simulink model "controllo_cartesiano"  (R2020b)
settings: Solver=VariableStepAuto  StartTime=0.0  StopTime=10.0  RelTol=1e-3
values from neighbouring files (symbols this model uses):
  f_G1 =     [workspaceMassaGravitaCoriolis.mat]
  f_G2 =     [workspaceMassaGravitaCoriolis.mat]
  f_G3 =     [workspaceMassaGravitaCoriolis.mat]
  f_M11 =     [workspaceMassaGravitaCoriolis.mat]
  f_M12 =     [workspaceMassaGravitaCoriolis.mat]
  f_M13 =     [workspaceMassaGravitaCoriolis.mat]
  f_M21 =     [workspaceMassaGravitaCoriolis.mat]
  f_M22 =     [workspaceMassaGravitaCoriolis.mat]
  f_M23 =     [workspaceMassaGravitaCoriolis.mat]
  f_M31 =     [workspaceMassaGravitaCoriolis.mat]
  f_M32 =     [workspaceMassaGravitaCoriolis.mat]
  f_M33 =     [workspaceMassaGravitaCoriolis.mat]
  f_V1 =     [workspaceMassaGravitaCoriolis.mat]
  f_V2 =     [workspaceMassaGravitaCoriolis.mat]
  f_V3 =     [workspaceMassaGravitaCoriolis.mat]
libraries: robotcorelib x1
(part 1 of 5)
settings Model: Creator=frasi  LastModifiedBy=frasi

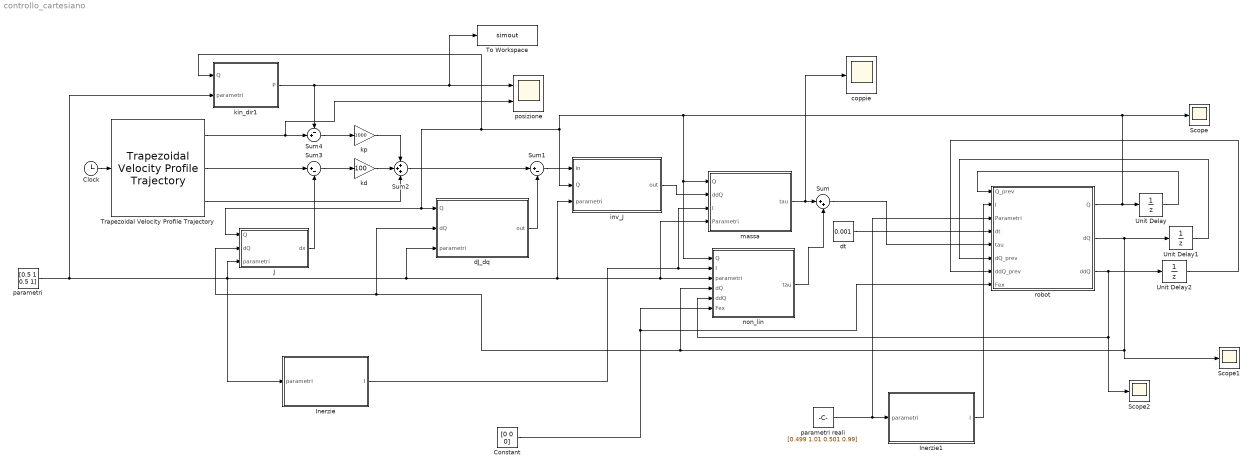
== system controllo_cartesiano ==
  Clock : Clock
  Constant : Constant  Value=[0 0 0]
  Inerzie : MATLAB Function  TreatAsAtomicUnit=on
  Inerzie1 : MATLAB Function  TreatAsAtomicUnit=on
  J : MATLAB Function  TreatAsAtomicUnit=on
  Scope : Scope
  Scope1 : Scope
  Scope2 : Scope
  Sum : Sum  Inputs=|++
  Sum1 : Sum  Inputs=|+-
  Sum2 : Sum  Inputs=+++
  Sum3 : Sum  Inputs=|+-
  Sum4 : Sum  Inputs=-+|
  To Workspace : ToWorkspace  VariableName=simout  SaveFormat=Timeseries  SampleTime=-1
  Trapezoidal Velocity Profile Trajectory : robotcorelib/Trapezoidal Velocity Profile Trajectory  WaypointSource=Internal  Waypoints=[1 1.5; 1.5 2;pi/6 pi/4]  NumParams=1  Parameter1=End Time  Parameter2=Peak Velocity  ParameterSource=Internal  PeakVelocity=[ 4;4 ]  Acceleration=[ 8; 8 ]  EndTime=[ 1; 1 ]  AccelTime=[ 1; 2 ]  SimulateUsing=Interpreted execution
      settings: SourceProductBaseCode=NV,RO,RR,UV
  Unit Delay : UnitDelay  InitialCondition="[0.2403    2.6314    0.9562]"  SampleTime=-1  HasFrameUpgradeWarning=on
  Unit Delay1 : UnitDelay  InitialCondition=[0 0 0]  SampleTime=-1  HasFrameUpgradeWarning=on
  Unit Delay2 : UnitDelay  InitialCondition=[0 0 0]  SampleTime=-1  HasFrameUpgradeWarning=on
  coppie : Scope
  dJ_dq : MATLAB Function  TreatAsAtomicUnit=on
  dt : Constant  Value=0.001
  inv_J : MATLAB Function  TreatAsAtomicUnit=on
  kd : Gain  Gain=100
  kin_dir1 : MATLAB Function  TreatAsAtomicUnit=on
  kp : Gain  Gain=1000
  massa : Subsystem
  non_lin : Subsystem
  parametri : Constant  Value=[0.5 1 0.5 1]
  parametri reali : Constant  Value=[0.499 1.01 0.501 0.99]
  posizione : Scope  NumInputPorts=2
  robot : Subsystem
  wires:
  Trapezoidal Velocity Profile Trajectory/3 -> Sum2/3
  Sum/1 -> robot/5(tau)
  dt/1 -> robot/4(dt)
  kp/1 -> Sum2/1
  Sum3/1 -> kd/1
  Trapezoidal Velocity Profile Trajectory/2 -> Sum3/1
  Sum4/1 -> kp/1
  J/1(dx) -> Sum3/2
  kin_dir1/1(P) -> Sum4/1, To Workspace/1, posizione/1
  Sum1/1 -> inv_J/1(in)
  Sum2/1 -> Sum1/1
  robot/2(dQ) -> Unit Delay1/1, Scope1/1, non_lin/4(dQ), J/2(dQ), dJ_dq/2(dQ)
  non_lin/1(tau) -> Sum/2
  parametri reali/1 -> Inerzie1/1(parametri), robot/3(Parametri)
  parametri/1 -> kin_dir1/2(parametri), inv_J/3(parametri), massa/4(Parametri), non_lin/3(parametri), dJ_dq/3(parametri), Inerzie/1(parametri), J/3(parametri)
  Trapezoidal Velocity Profile Trajectory/1 -> posizione/2, Sum4/2
  kd/1 -> Sum2/2
  massa/1(tau) -> coppie/1, Sum/1
  robot/1(Q) -> non_lin/1(Q), massa/1(Q), kin_dir1/1(Q), J/1(Q), dJ_dq/1(Q), inv_J/2(Q), Scope/1, Unit Delay/1
  Clock/1 -> Trapezoidal Velocity Profile Trajectory/1
  dJ_dq/1(out) -> Sum1/2
  Unit Delay/1 -> robot/1(Q_prev)
  Unit Delay1/1 -> robot/6(dQ_prev)
  inv_J/1(out) -> massa/2(ddQ)
  robot/3(ddQ) -> Unit Delay2/1, Scope2/1, non_lin/5(ddQ)
  Unit Delay2/1 -> robot/7(ddQ_prev)
  Inerzie/1(I) -> massa/3(I), non_lin/2(I)
  Inerzie1/1(I) -> robot/2(I)
  Constant/1 -> non_lin/6(Fex), robot/8(Fex)

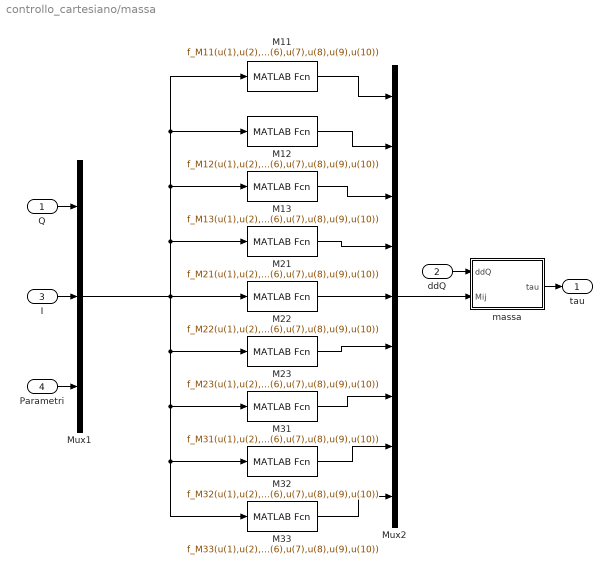
== system controllo_cartesiano/massa ==
  Q : Inport
  ddQ : Inport  Port=2
  I : Inport  Port=3
  Parametri : Inport  Port=4
  M11 : MATLABFcn  MATLABFcn=f_M11(u(1),u(2),u(3),u(4),u(5),u(6),u(7),u(8),u(9),u(10))
  M12 : MATLABFcn  MATLABFcn=f_M12(u(1),u(2),u(3),u(4),u(5),u(6),u(7),u(8),u(9),u(10))
  M13 : MATLABFcn  MATLABFcn=f_M13(u(1),u(2),u(3),u(4),u(5),u(6),u(7),u(8),u(9),u(10))
  M21 : MATLABFcn  MATLABFcn=f_M21(u(1),u(2),u(3),u(4),u(5),u(6),u(7),u(8),u(9),u(10))
  M22 : MATLABFcn  MATLABFcn=f_M22(u(1),u(2),u(3),u(4),u(5),u(6),u(7),u(8),u(9),u(10))
  M23 : MATLABFcn  MATLABFcn=f_M23(u(1),u(2),u(3),u(4),u(5),u(6),u(7),u(8),u(9),u(10))
  M31 : MATLABFcn  MATLABFcn=f_M31(u(1),u(2),u(3),u(4),u(5),u(6),u(7),u(8),u(9),u(10))
  M32 : MATLABFcn  MATLABFcn=f_M32(u(1),u(2),u(3),u(4),u(5),u(6),u(7),u(8),u(9),u(10))
  M33 : MATLABFcn  MATLABFcn=f_M33(u(1),u(2),u(3),u(4),u(5),u(6),u(7),u(8),u(9),u(10))
  Mux1 : Mux  Inputs=3
  Mux2 : Mux  Inputs=9
  massa : MATLAB Function  TreatAsAtomicUnit=on
  tau : Outport
  wires:
  M13/1 -> Mux2/3
  Mux2/1 -> massa/2(Mij)
  M33/1 -> Mux2/9
  M11/1 -> Mux2/1
  Mux1/1 -> M13/1, M12/1, M11/1, M21/1, M31/1, M32/1, M33/1, M23/1, M22/1
  M22/1 -> Mux2/5
  M23/1 -> Mux2/6
  M31/1 -> Mux2/7
  M21/1 -> Mux2/4
  M12/1 -> Mux2/2
  Parametri/1 -> Mux1/3
  M32/1 -> Mux2/8
  ddQ/1 -> massa/1(ddQ)
  I/1 -> Mux1/2
  Q/1 -> Mux1/1
  massa/1(tau) -> tau/1

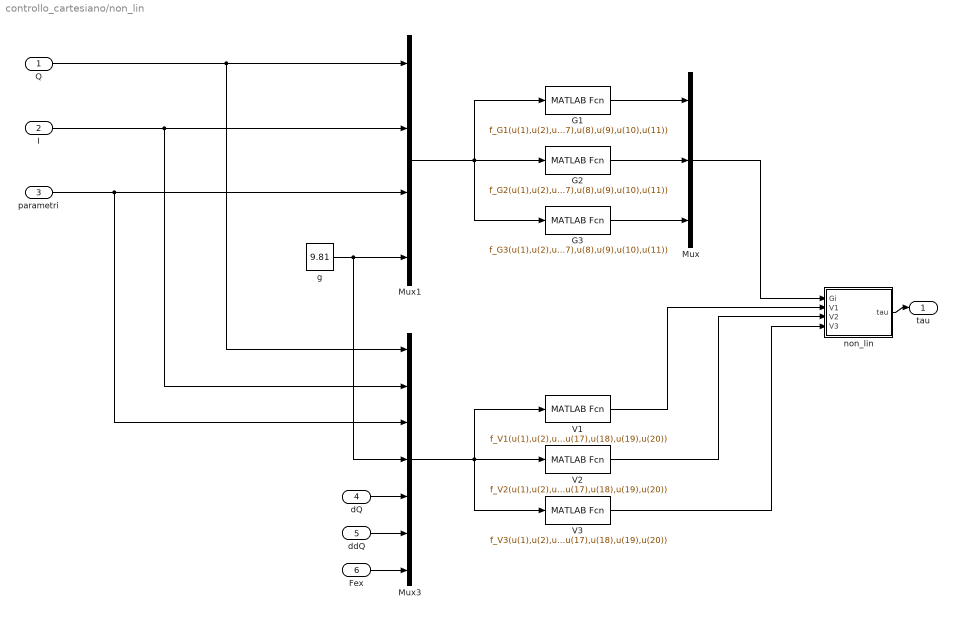
== system controllo_cartesiano/non_lin ==
  Q : Inport
  I : Inport  Port=2
  parametri : Inport  Port=3
  dQ : Inport  Port=4
  ddQ : Inport  Port=5
  Fex : Inport  Port=6
  G1 : MATLABFcn  MATLABFcn=f_G1(u(1),u(2),u(3),u(4),u(5),u(6),u(7),u(8),u(9),u(10),u(11))
  G2 : MATLABFcn  MATLABFcn=f_G2(u(1),u(2),u(3),u(4),u(5),u(6),u(7),u(8),u(9),u(10),u(11))
  G3 : MATLABFcn  MATLABFcn=f_G3(u(1),u(2),u(3),u(4),u(5),u(6),u(7),u(8),u(9),u(10),u(11))
  Mux : Mux  Inputs=3
  Mux1 : Mux
  Mux3 : Mux  Inputs=7
  V1 : MATLABFcn  MATLABFcn=f_V1(u(1),u(2),u(3),u(4),u(5),u(6),u(7),u(8),u(9),u(10),u(11),u(12),u(13),u(14),u(15),u(16),u(17),u(18),u(19),u(20))
  V2 : MATLABFcn  MATLABFcn=f_V2(u(1),u(2),u(3),u(4),u(5),u(6),u(7),u(8),u(9),u(10),u(11),u(12),u(13),u(14),u(15),u(16),u(17),u(18),u(19),u(20))
  V3 : MATLABFcn  MATLABFcn=f_V3(u(1),u(2),u(3),u(4),u(5),u(6),u(7),u(8),u(9),u(10),u(11),u(12),u(13),u(14),u(15),u(16),u(17),u(18),u(19),u(20))
  g : Constant  Value=9.81
  non_lin : MATLAB Function  TreatAsAtomicUnit=on
  tau : Outport
  wires:
  Mux3/1 -> V3/1, V2/1, V1/1
  g/1 -> Mux3/4, Mux1/4
  parametri/1 -> Mux3/3, Mux1/3
  Mux1/1 -> G3/1, G2/1, G1/1
  non_lin/1(tau) -> tau/1
  Q/1 -> Mux3/1, Mux1/1
  Fex/1 -> Mux3/7
  I/1 -> Mux3/2, Mux1/2
  dQ/1 -> Mux3/5
  ddQ/1 -> Mux3/6
  V1/1 -> non_lin/2(V1)
  V2/1 -> non_lin/3(V2)
  V3/1 -> non_lin/4(V3)
  Mux/1 -> non_lin/1(Gi)
  G1/1 -> Mux/1
  G2/1 -> Mux/2
  G3/1 -> Mux/3

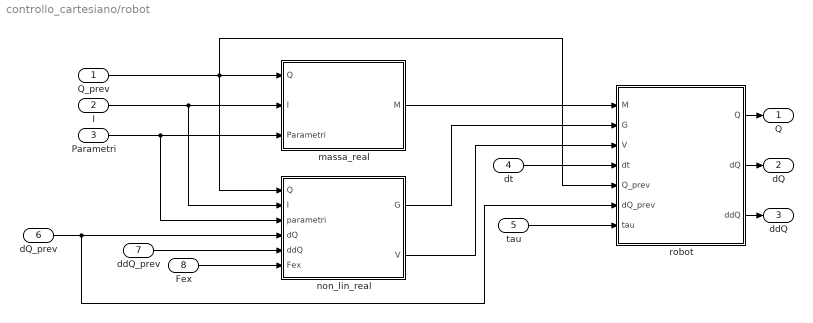
== system controllo_cartesiano/robot ==
  Q_prev : Inport
  I : Inport  Port=2
  Parametri : Inport  Port=3
  dt : Inport  Port=4
  tau : Inport  Port=5
  dQ_prev : Inport  Port=6
  ddQ_prev : Inport  Port=7
  Fex : Inport  Port=8
  massa_real : Subsystem
  non_lin_real : Subsystem
  robot : MATLAB Function  TreatAsAtomicUnit=on
  Q : Outport
  dQ : Outport  Port=2
  ddQ : Outport  Port=3
  wires:
  Parametri/1 -> non_lin_real/3(parametri), massa_real/3(Parametri)
  non_lin_real/1(G) -> robot/2(G)
  ddQ_prev/1 -> non_lin_real/5(ddQ)
  Fex/1 -> non_lin_real/6(Fex)
  non_lin_real/2(V) -> robot/3(V)
  I/1 -> non_lin_real/2(I), massa_real/2(I)
  massa_real/1(M) -> robot/1(M)
  robot/1(Q) -> Q/1
  Q_prev/1 -> robot/5(Q_prev), massa_real/1(Q), non_lin_real/1(Q)
  dQ_prev/1 -> robot/6(dQ_prev), non_lin_real/4(dQ)
  tau/1 -> robot/7(tau)
  robot/2(dQ) -> dQ/1
  dt/1 -> robot/4(dt)
  robot/3(ddQ) -> ddQ/1

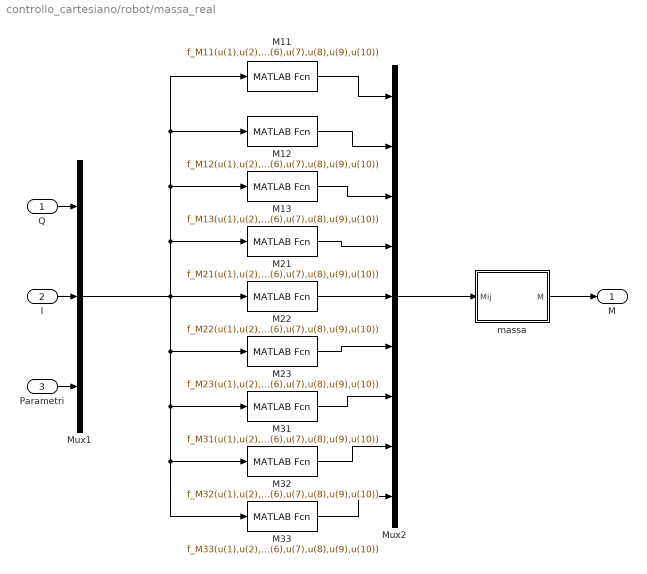
== system controllo_cartesiano/robot/massa_real ==
  Q : Inport
  I : Inport  Port=2
  Parametri : Inport  Port=3
  M11 : MATLABFcn  MATLABFcn=f_M11(u(1),u(2),u(3),u(4),u(5),u(6),u(7),u(8),u(9),u(10))
  M12 : MATLABFcn  MATLABFcn=f_M12(u(1),u(2),u(3),u(4),u(5),u(6),u(7),u(8),u(9),u(10))
  M13 : MATLABFcn  MATLABFcn=f_M13(u(1),u(2),u(3),u(4),u(5),u(6),u(7),u(8),u(9),u(10))
  M21 : MATLABFcn  MATLABFcn=f_M21(u(1),u(2),u(3),u(4),u(5),u(6),u(7),u(8),u(9),u(10))
  M22 : MATLABFcn  MATLABFcn=f_M22(u(1),u(2),u(3),u(4),u(5),u(6),u(7),u(8),u(9),u(10))
  M23 : MATLABFcn  MATLABFcn=f_M23(u(1),u(2),u(3),u(4),u(5),u(6),u(7),u(8),u(9),u(10))
  M31 : MATLABFcn  MATLABFcn=f_M31(u(1),u(2),u(3),u(4),u(5),u(6),u(7),u(8),u(9),u(10))
  M32 : MATLABFcn  MATLABFcn=f_M32(u(1),u(2),u(3),u(4),u(5),u(6),u(7),u(8),u(9),u(10))
  M33 : MATLABFcn  MATLABFcn=f_M33(u(1),u(2),u(3),u(4),u(5),u(6),u(7),u(8),u(9),u(10))
  Mux1 : Mux  Inputs=3
  Mux2 : Mux  Inputs=9
  massa : MATLAB Function  TreatAsAtomicUnit=on
  M : Outport
  wires:
  M13/1 -> Mux2/3
  Mux2/1 -> massa/1(Mij)
  M33/1 -> Mux2/9
  M11/1 -> Mux2/1
  Mux1/1 -> M13/1, M12/1, M11/1, M21/1, M31/1, M32/1, M33/1, M23/1, M22/1
  M22/1 -> Mux2/5
  M23/1 -> Mux2/6
  M31/1 -> Mux2/7
  M21/1 -> Mux2/4
  M12/1 -> Mux2/2
  Parametri/1 -> Mux1/3
  M32/1 -> Mux2/8
  I/1 -> Mux1/2
  Q/1 -> Mux1/1
  massa/1(M) -> M/1

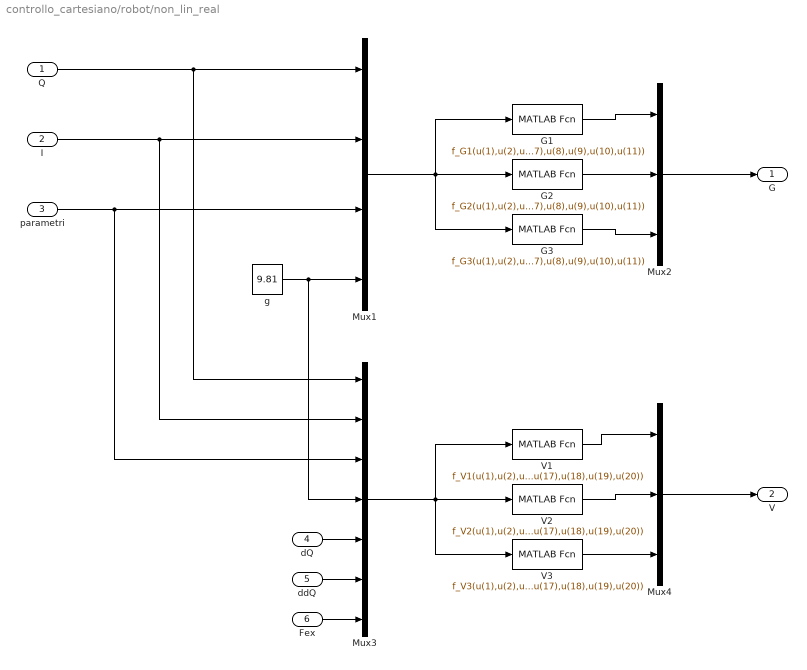
== system controllo_cartesiano/robot/non_lin_real ==
  Q : Inport
  I : Inport  Port=2
  parametri : Inport  Port=3
  dQ : Inport  Port=4
  ddQ : Inport  Port=5
  Fex : Inport  Port=6
  G1 : MATLABFcn  MATLABFcn=f_G1(u(1),u(2),u(3),u(4),u(5),u(6),u(7),u(8),u(9),u(10),u(11))
  G2 : MATLABFcn  MATLABFcn=f_G2(u(1),u(2),u(3),u(4),u(5),u(6),u(7),u(8),u(9),u(10),u(11))
  G3 : MATLABFcn  MATLABFcn=f_G3(u(1),u(2),u(3),u(4),u(5),u(6),u(7),u(8),u(9),u(10),u(11))
  Mux1 : Mux
  Mux2 : Mux  Inputs=3
  Mux3 : Mux  Inputs=7
  Mux4 : Mux  Inputs=3
  V1 : MATLABFcn  MATLABFcn=f_V1(u(1),u(2),u(3),u(4),u(5),u(6),u(7),u(8),u(9),u(10),u(11),u(12),u(13),u(14),u(15),u(16),u(17),u(18),u(19),u(20))
  V2 : MATLABFcn  MATLABFcn=f_V2(u(1),u(2),u(3),u(4),u(5),u(6),u(7),u(8),u(9),u(10),u(11),u(12),u(13),u(14),u(15),u(16),u(17),u(18),u(19),u(20))
  V3 : MATLABFcn  MATLABFcn=f_V3(u(1),u(2),u(3),u(4),u(5),u(6),u(7),u(8),u(9),u(10),u(11),u(12),u(13),u(14),u(15),u(16),u(17),u(18),u(19),u(20))
  g : Constant  Value=9.81
  G : Outport
  V : Outport  Port=2
  wires:
  Mux3/1 -> V3/1, V2/1, V1/1
  g/1 -> Mux3/4, Mux1/4
  V2/1 -> Mux4/2
  G2/1 -> Mux2/2
  Q/1 -> Mux3/1, Mux1/1
  Mux1/1 -> G3/1, G2/1, G1/1
  V3/1 -> Mux4/3
  V1/1 -> Mux4/1
  G1/1 -> Mux2/1
  G3/1 -> Mux2/3
  Mux4/1 -> V/1
  Mux2/1 -> G/1
  parametri/1 -> Mux3/3, Mux1/3
  Fex/1 -> Mux3/7
  I/1 -> Mux3/2, Mux1/2
  ddQ/1 -> Mux3/6
  dQ/1 -> Mux3/5

== matlab function controllo_cartesiano/non_lin/non_lin ==
  data: Gi input; tau output; V1 input; V2 input; V3 input
function tau = non_lin(Gi,V1,V2,V3)

G=[Gi(1);Gi(2);Gi(3)];
V=[V1;V2;V3];

tau=G+V;
end

== matlab function controllo_cartesiano/massa/massa ==
  data: ddQ input; tau output; Mij input
function  tau= massa(ddQ,Mij)

M=[Mij(1) Mij(2) Mij(3);Mij(4) Mij(5) Mij(6);Mij(7) Mij(8) Mij(9)];
tau=M*ddQ;

end

== matlab function controllo_cartesiano/inv_J ==
  data: in input; out output; Q input; parametri input
function out = inv_J(in,Q,parametri)
l=parametri(1);
d=parametri(2);
% m1=parametri(3);
% ma=parametri(4);
xc1=Q(1);
xc5=Q(2);
q2=Q(3);

J =[...
 
(l*sin(2*atan((2*l^2*sin(q2) + (3*l^4 + 4*cos(q2)*l^3*xc1 - 4*sin(q2)*l^3*xc5 - 2*cos(2*q2)*l^2*xc1^2 + 4*sin(2*q2)*l^2*xc1*xc5 + 2*cos(2*q2)*l^2*xc5^2 - 4*cos(q2)*l*xc1^3 + 4*sin(q2)*l*xc1^2*xc5 - 4*cos(q2)*l*xc1*xc5^2 + 4*sin(q2)*l*xc5^3 - xc1^4 - 2*xc1^2*xc5^2 - xc5^4)^(1/2) - 2*l*xc5)/(l^2 - 2*l*xc1 + xc1^2 + xc5^2 - 2*l^2*cos(q2) + 2*l*xc1*cos(q2) - 2*l*xc5*sin(q2))))*(((2*xc1 - 2*l + 2*l*cos(q2))*(2*l^2*sin(q2) + (3*l^4 + 4*cos(q2)*l^3*xc1 - 4*sin(q2)*l^3*xc5 - 2*cos(2*q2)*l^2*xc1^2 + 4*sin(2*q2)*l^2*xc1*xc5 + 2*cos(2*q2)*l^2*xc5^2 - 4*cos(q2)*l*xc1^3 + 4*sin(q2)*l*xc1^2*xc5 - 4*cos(q2)*l*xc1*xc5^2 + 4*sin(q2)*l*xc5^3 - xc1^4 - 2*xc1^2*xc5^2 - xc5^4)^(1/2) - 2*l*xc5))/(l^2 - 2*l*xc1 + xc1^2 + xc5^2 - 2*l^2*cos(q2) + 2*l*xc1*cos(q2) - 2*l*xc5*sin(q2))^2 + (2*(xc1 + l*cos(q2))*(- l^2 + 2*cos(q2)*l*xc1 - 2*sin(q2)*l*xc5 + xc1^2 + xc5^2))/((l^2 - 2*l*xc1 + xc1^2 + xc5^2 - 2*l^2*cos(q2) + 2*l*xc1*cos(q2) - 2*l*xc5*sin(q2))*(3*l^4 + 4*cos(q2)*l^3*xc1 - 4*sin(q2)*l^3*xc5 - 2*cos(2*q2)*l^2*xc1^2 + 4*sin(2*q2)*l^2*xc1*xc5 + 2*cos(2*q2)*l^2*xc5^2 - 4*cos(q2)*l*xc1^3 + 4*sin(q2)*l*xc1^2*xc5 - 4*cos(q2)*l*xc1*xc5^2 + 4*sin(q2)*l*xc5^3 - xc1^4 - 2*xc1^2*xc5^2 - xc5^4)^(1/2))))/((2*l^2*sin(q2) + (3*l^4 + 4*cos(q2)*l^3*xc1 - 4*sin(q2)*l^3*xc5 - 2*cos(2*q2)*l^2*xc1^2 + 4*sin(2*q2)*l^2*xc1*xc5 + 2*cos(2*q2)*l^2*xc5^2 - 4*cos(q2)*l*xc1^3 + 4*sin(q2)*l*xc1^2*xc5 - 4*cos(q2)*l*xc1*xc5^2 + 4*sin(q2)*l*xc5^3 - xc1^4 - 2*xc1^2*xc5^2 - xc5^4)^(1/2) - 2*l*xc5)^2/(l^2 - 2*l*xc1 + xc1^2 + xc5^2 - 2*l^2*cos(q2) + 2*l*xc1*cos(q2) - 2*l*xc5*sin(q2))^2 + 1) + 1, (l*sin(2*atan((2*l^2*sin(q2) + (3*l^4 + 4*cos(q2)*l^3*xc1 - 4*sin(q2)*l^3*xc5 - 2*cos(2*q2)*l^2*xc1^2 + 4*sin(2*q2)*l^2*xc1*xc5 + 2*cos(2*q2)*l^2*xc5^2 - 4*cos(q2)*l*xc1^3 + 4*sin(q2)*l*xc1^2*xc5 - 4*cos(q2)*l*xc1*xc5^2 + 4*sin(q2)*l*xc5^3 - xc1^4 - 2*xc1^2*xc5^2 - xc5^4)^(1/2) - 2*l*xc5)/(l^2 - 2*l*xc1 + xc1^2 + xc5^2 - 2*l^2*cos(q2) + 2*l*xc1*cos(q2) - 2*l*xc5*sin(q2))))*((2*l + (2*sin(q2)*l^3 - 2*sin(2*q2)*l^2*xc1 - 2*cos(2*q2)*l^2*xc5 - 2*sin(q2)*l*xc1^2 + 4*cos(q2)*l*xc1*xc5 - 6*sin(q2)*l*xc5^2 + 2*xc1^2*xc5 + 2*xc5^3)/(3*l^4 + 4*cos(q2)*l^3*xc1 - 4*sin(q2)*l^3*xc5 - 2*cos(2*q2)*l^2*xc1^2 + 4*sin(2*q2)*l^2*xc1*xc5 + 2*cos(2*q2)*l^2*xc5^2 - 4*cos(q2)*l*xc1^3 + 4*sin(q2)*l*xc1^2*xc5 - 4*cos(q2)*l*xc1*xc5^2 + 4*sin(q2)*l*xc5^3 - xc1^4 - 2*xc1^2*xc5^2 - xc5^4)^(1/2))/(l^2 - 2*l*xc1 + xc1^2 + xc5^2 - 2*l^2*cos(q2) + 2*l*xc1*cos(q2) - 2*l*xc5*sin(q2)) + ((2*xc5 - 2*l*sin(q2))*(2*l^2*sin(q2) + (3*l^4 + 4*cos(q2)*l^3*xc1 - 4*sin(q2)*l^3*xc5 - 2*cos(2*q2)*l^2*xc1^2 + 4*sin(2*q2)*l^2*xc1*xc5 + 2*cos(2*q2)*l^2*xc5^2 - 4*cos(q2)*l*xc1^3 + 4*sin(q2)*l*xc1^2*xc5 - 4*cos(q2)*l*xc1*xc5^2 + 4*sin(q2)*l*xc5^3 - xc1^4 - 2*xc1^2*xc5^2 - xc5^4)^(1/2) - 2*l*xc5))/(l^2 - 2*l*xc1 + xc1^2 + xc5^2 - 2*l^2*cos(q2) + 2*l*xc1*cos(q2) - 2*l*xc5*sin(q2))^2))/((2*l^2*sin(q2) + (3*l^4 + 4*cos(q2)*l^3*xc1 - 4*sin(q2)*l^3*xc5 - 2*cos(2*q2)*l^2*xc1^2 + 4*sin(2*q2)*l^2*xc1*xc5 + 2*cos(2*q2)*l^2*xc5^2 - 4*cos(q2)*l*xc1^3 + 4*sin(q2)*l*xc1^2*xc5 - 4*cos(q2)*l*xc1*xc5^2 + 4*sin(q2)*l*xc5^3 - xc1^4 - 2*xc1^2*xc5^2 - xc5^4)^(1/2) - 2*l*xc5)^2/(l^2 - 2*l*xc1 + xc1^2 + xc5^2 - 2*l^2*cos(q2) + 2*l*xc1*cos(q2) - 2*l*xc5*sin(q2))^2 + 1), - l*sin(q2) - (l*sin(2*atan((2*l^2*sin(q2) + (3*l^4 + 4*cos(q2)*l^3*xc1 - 4*sin(q2)*l^3*xc5 - 2*cos(2*q2)*l^2*xc1^2 + 4*sin(2*q2)*l^2*xc1*xc5 + 2*cos(2*q2)*l^2*xc5^2 - 4*cos(q2)*l*xc1^3 + 4*sin(q2)*l*xc1^2*xc5 - 4*cos(q2)*l*xc1*xc5^2 + 4*sin(q2)*l*xc5^3 - xc1^4 - 2*xc1^2*xc5^2 - xc5^4)^(1/2) - 2*l*xc5)/(l^2 - 2*l*xc1 + xc1^2 + xc5^2 - 2*l^2*cos(q2) + 2*l*xc1*cos(q2) - 2*l*xc5*sin(q2))))*((2*l^2*cos(q2) + (2*l*(- sin(q2)*l^2*xc1 - cos(q2)*l^2*xc5 + sin(2*q2)*l*xc1^2 + 2*cos(2*q2)*l*xc1*xc5 - sin(2*q2)*l*xc5^2 + sin(q2)*xc1^3 + cos(q2)*xc1^2*xc5 + sin(q2)*xc1*xc5^2 + cos(q2)*xc5^3))/(3*l^4 + 4*cos(q2)*l^3*xc1 - 4*sin(q2)*l^3*xc5 - 2*cos(2*q2)*l^2*xc1^2 + 4*sin(2*q2)*l^2*xc1*xc5 + 2*cos(2*q2)*l^2*xc5^2 - 4*cos(q2)*l*xc1^3 + 4*sin(q2)*l*xc1^2*xc5 - 4*cos(q2)*l*xc1*xc5^2 + 4*sin(q2)*l*xc5^3 - xc1^4 - 2*xc1^2*xc5^2 - xc5^4)^(1/2))/(l^2 - 2*l*xc1 + xc1^2 + xc5^2 - 2*l^2*cos(q2) + 2*l*xc1*cos(q2) - 2*l*xc5*sin(q2)) + (2*l*(xc5*cos(q2) - l*sin(q2) + xc1*sin(q2))*(2*l^2*sin(q2) + (3*l^4 + 4*cos(q2)*l^3*xc1 - 4*sin(q2)*l^3*xc5 - 2*cos(2*q2)*l^2*xc1^2 + 4*sin(2*q2)*l^2*xc1*xc5 + 2*cos(2*q2)*l^2*xc5^2 - 4*cos(q2)*l*xc1^3 + 4*sin(q2)*l*xc1^2*xc5 - 4*cos(q2)*l*xc1*xc5^2 + 4*sin(q2)*l*xc5^3 - xc1^4 - 2*xc1^2*xc5^2 - xc5^4)^(1/2) - 2*l*xc5))/(l^2 - 2*l*xc1 + xc1^2 + xc5^2 - 2*l^2*cos(q2) + 2*l*xc1*cos(q2) - 2*l*xc5*sin(q2))^2))/((2*l^2*sin(q2) + (3*l^4 + 4*cos(q2)*l^3*xc1 - 4*sin(q2)*l^3*xc5 - 2*cos(2*q2)*l^2*xc1^2 + 4*sin(2*q2)*l^2*xc1*xc5 + 2*cos(2*q2)*l^2*xc5^2 - 4*cos(q2)*l*xc1^3 + 4*sin(q2)*l*xc1^2*xc5 - 4*cos(q2)*l*xc1*xc5^2 + 4*sin(q2)*l*xc5^3 - xc1^4 - 2*xc1^2*xc5^2 - xc5^4)^(1/2) - 2*l*xc5)^2/(l^2 - 2*l*xc1 + xc1^2 + xc5^2 - 2*l^2*cos(q2) + 2*l*xc1*cos(q2) - 2*l*xc5*sin(q2))^2 + 1);...
    (l*cos(2*atan((2*l^2*sin(q2) + (3*l^4 + 4*cos(q2)*l^3*xc1 - 4*sin(q2)*l^3*xc5 - 2*cos(2*q2)*l^2*xc1^2 + 4*sin(2*q2)*l^2*xc1*xc5 + 2*cos(2*q2)*l^2*xc5^2 - 4*cos(q2)*l*xc1^3 + 4*sin(q2)*l*xc1^2*xc5 - 4*cos(q2)*l*xc1*xc5^2 + 4*sin(q2)*l*xc5^3 - xc1^4 - 2*xc1^2*xc5^2 - xc5^4)^(1/2) - 2*l*xc5)/(l^2 - 2*l*xc1 + xc1^2 + xc5^2 - 2*l^2*cos(q2) + 2*l*xc1*cos(q2) - 2*l*xc5*sin(q2))))*(((2*xc1 - 2*l + 2*l*cos(q2))*(2*l^2*sin(q2) + (3*l^4 + 4*cos(q2)*l^3*xc1 - 4*sin(q2)*l^3*xc5 - 2*cos(2*q2)*l^2*xc1^2 + 4*sin(2*q2)*l^2*xc1*xc5 + 2*cos(2*q2)*l^2*xc5^2 - 4*cos(q2)*l*xc1^3 + 4*sin(q2)*l*xc1^2*xc5 - 4*cos(q2)*l*xc1*xc5^2 + 4*sin(q2)*l*xc5^3 - xc1^4 - 2*xc1^2*xc5^2 - xc5^4)^(1/2) - 2*l*xc5))/(l^2 - 2*l*xc1 + xc1^2 + xc5^2 - 2*l^2*cos(q2) + 2*l*xc1*cos(q2) - 2*l*xc5*sin(q2))^2 + (2*(xc1 + l*cos(q2))*(- l^2 + 2*cos(q2)*l*xc1 - 2*sin(q2)*l*xc5 + xc1^2 + xc5^2))/((l^2 - 2*l*xc1 + xc1^2 + xc5^2 - 2*l^2*cos(q2) + 2*l*xc1*cos(q2) - 2*l*xc5*sin(q2))*(3*l^4 + 4*cos(q2)*l^3*xc1 - 4*sin(q2)*l^3*xc5 - 2*cos(2*q2)*l^2*xc1^2 + 4*sin(2*q2)*l^2*xc1*xc5 + 2*cos(2*q2)*l^2*xc5^2 - 4*cos(q2)*l*xc1^3 + 4*sin(q2)*l*xc1^2*xc5 - 4*cos(q2)*l*xc1*xc5^2 + 4*sin(q2)*l*xc5^3 - xc1^4 - 2*xc1^2*xc5^2 - xc5^4)^(1/2))))/((2*l^2*sin(q2) + (3*l^4 + 4*cos(q2)*l^3*xc1 - 4*sin(q2)*l^3*xc5 - 2*cos(2*q2)*l^2*xc1^2 + 4*sin(2*q2)*l^2*xc1*xc5 + 2*cos(2*q2)*l^2*xc5^2 - 4*cos(q2)*l*xc1^3 + 4*sin(q2)*l*xc1^2*xc5 - 4*cos(q2)*l*xc1*xc5^2 + 4*sin(q2)*l*xc5^3 - xc1^4 - 2*xc1^2*xc5^2 - xc5^4)^(1/2) - 2*l*xc5)^2/(l^2 - 2*l*xc1 + xc1^2 + xc5^2 - 2*l^2*cos(q2) + 2*l*xc1*cos(q2) - 2*l*xc5*sin(q2))^2 + 1), (l*cos(2*atan((2*l^2*sin(q2) + (3*l^4 + 4*cos(q2)*l^3*xc1 - 4*sin(q2)*l^3*xc5 - 2*cos(2*q2)*l^2*xc1^2 + 4*sin(2*q2)*l^2*xc1*xc5 + 2*cos(2*q2)*l^2*xc5^2 - 4*cos(q2)*l*xc1^3 + 4*sin(q2)*l*xc1^2*xc5 - 4*cos(q2)*l*xc1*xc5^2 + 4*sin(q2)*l*xc5^3 - xc1^4 - 2*xc1^2*xc5^2 - xc5^4)^(1/2) - 2*l*xc5)/(l^2 - 2*l*xc1 + xc1^2 + xc5^2 - 2*l^2*cos(q2) + 2*l*xc1*cos(q2) - 2*l*xc5*sin(q2))))*((2*l + (2*sin(q2)*l^3 - 2*sin(2*q2)*l^2*xc1 - 2*cos(2*q2)*l^2*xc5 - 2*sin(q2)*l*xc1^2 + 4*cos(q2)*l*xc1*xc5 - 6*sin(q2)*l*xc5^2 + 2*xc1^2*xc5 + 2*xc5^3)/(3*l^4 + 4*cos(q2)*l^3*xc1 - 4*sin(q2)*l^3*xc5 - 2*cos(2*q2)*l^2*xc1^2 + 4*sin(2*q2)*l^2*xc1*xc5 + 2*cos(2*q2)*l^2*xc5^2 - 4*cos(q2)*l*xc1^3 + 4*sin(q2)*l*xc1^2*xc5 - 4*cos(q2)*l*xc1*xc5^2 + 4*sin(q2)*l*xc5^3 - xc1^4 - 2*xc1^2*xc5^2 - xc5^4)^(1/2))/(l^2 - 2*l*xc1 + xc1^2 + xc5^2 - 2*l^2*cos(q2) + 2*l*xc1*cos(q2) - 2*l*xc5*sin(q2)) + ((2*xc5 - 2*l*sin(q2))*(2*l^2*sin(q2) + (3*l^4 + 4*cos(q2)*l^3*xc1 - 4*sin(q2)*l^3*xc5 - 2*cos(2*q2)*l^2*xc1^2 + 4*sin(2*q2)*l^2*xc1*xc5 + 2*cos(2*q2)*l^2*xc5^2 - 4*cos(q2)*l*xc1^3 + 4*sin(q2)*l*xc1^2*xc5 - 4*cos(q2)*l*xc1*xc5^2 + 4*sin(q2)*l*xc5^3 - xc1^4 - 2*xc1^2*xc5^2 - xc5^4)^(1/2) - 2*l*xc5))/(l^2 - 2*l*xc1 + xc1^2 + xc5^2 - 2*l^2*cos(q2) + 2*l*xc1*cos(q2) - 2*l*xc5*sin(q2))^2))/((2*l^2*sin(q2) + (3*l^4 + 4*cos(q2)*l^3*xc1 - 4*sin(q2)*l^3*xc5 - 2*cos(2*q2)*l^2*xc1^2 + 4*sin(2*q2)*l^2*xc1*xc5 + 2*cos(2*q2)*l^2*xc5^2 - 4*cos(q2)*l*xc1^3 + 4*sin(q2)*l*xc1^2*xc5 - 4*cos(q2)*l*xc1*xc5^2 + 4*sin(q2)*l*xc5^3 - xc1^4 - 2*xc1^2*xc5^2 - xc5^4)^(1/2) - 2*l*xc5)^2/(l^2 - 2*l*xc1 + xc1^2 + xc5^2 - 2*l^2*cos(q2) + 2*l*xc1*cos(q2) - 2*l*xc5*sin(q2))^2 + 1),   l*cos(q2) - (l*cos(2*atan((2*l^2*sin(q2) + (3*l^4 + 4*cos(q2)*l^3*xc1 - 4*sin(q2)*l^3*xc5 - 2*cos(2*q2)*l^2*xc1^2 + 4*sin(2*q2)*l^2*xc1*xc5 + 2*cos(2*q2)*l^2*xc5^2 - 4*cos(q2)*l*xc1^3 + 4*sin(q2)*l*xc1^2*xc5 - 4*cos(q2)*l*xc1*xc5^2 + 4*sin(q2)*l*xc5^3 - xc1^4 - 2*xc1^2*xc5^2 - xc5^4)^(1/2) - 2*l*xc5)/(l^2 - 2*l*xc1 + xc1^2 + xc5^2 - 2*l^2*cos(q2) + 2*l*xc1*cos(q2) - 2*l*xc5*sin(q2))))*((2*l^2*cos(q2) + (2*l*(- sin(q2)*l^2*xc1 - cos(q2)*l^2*xc5 + sin(2*q2)*l*xc1^2 + 2*cos(2*q2)*l*xc1*xc5 - sin(2*q2)*l*xc5^2 + sin(q2)*xc1^3 + cos(q2)*xc1^2*xc5 + sin(q2)*xc1*xc5^2 + cos(q2)*xc5^3))/(3*l^4 + 4*cos(q2)*l^3*xc1 - 4*sin(q2)*l^3*xc5 - 2*cos(2*q2)*l^2*xc1^2 + 4*sin(2*q2)*l^2*xc1*xc5 + 2*cos(2*q2)*l^2*xc5^2 - 4*cos(q2)*l*xc1^3 + 4*sin(q2)*l*xc1^2*xc5 - 4*cos(q2)*l*xc1*xc5^2 + 4*sin(q2)*l*xc5^3 - xc1^4 - 2*xc1^2*xc5^2 - xc5^4)^(1/2))/(l^2 - 2*l*xc1 + xc1^2 + xc5^2 - 2*l^2*cos(q2) + 2*l*xc1*cos(q2) - 2*l*xc5*sin(q2)) + (2*l*(xc5*cos(q2) - l*sin(q2) + xc1*sin(q2))*(2*l^2*sin(q2) + (3*l^4 + 4*cos(q2)*l^3*xc1 - 4*sin(q2)*l^3*xc5 - 2*cos(2*q2)*l^2*xc1^2 + 4*sin(2*q2)*l^2*xc1*xc5 + 2*cos(2*q2)*l^2*xc5^2 - 4*cos(q2)*l*xc1^3 + 4*sin(q2)*l*xc1^2*xc5 - 4*cos(q2)*l*xc1*xc5^2 + 4*sin(q2)*l*xc5^3 - xc1^4 - 2*xc1^2*xc5^2 - xc5^4)^(1/2) - 2*l*xc5))/(l^2 - 2*l*xc1 + xc1^2 + xc5^2 - 2*l^2*cos(q2) + 2*l*xc1*cos(q2) - 2*l*xc5*sin(q2))^2))/((2*l^2*sin(q2) + (3*l^4 + 4*cos(q2)*l^3*xc1 - 4*sin(q2)*l^3*xc5 - 2*cos(2*q2)*l^2*xc1^2 + 4*sin(2*q2)*l^2*xc1*xc5 + 2*cos(2*q2)*l^2*xc5^2 - 4*cos(q2)*l*xc1^3 + 4*sin(q2)*l*xc1^2*xc5 - 4*cos(q2)*l*xc1*xc5^2 + 4*sin(q2)*l*xc5^3 - xc1^4 - 2*xc1^2*xc5^2 - xc5^4)^(1/2) - 2*l*xc5)^2/(l^2 - 2*l*xc1 + xc1^2 + xc5^2 - 2*l^2*cos(q2) + 2*l*xc1*cos(q2) - 2*l*xc5*sin(q2))^2 + 1);...
                                                                                                                                                                                                                                                                                                                                                                                         (2*(((2*xc1 - 2*l + 2*l*cos(q2))*(2*l^2*sin(q2) + (3*l^4 + 4*cos(q2)*l^3*xc1 - 4*sin(q2)*l^3*xc5 - 2*cos(2*q2)*l^2*xc1^2 + 4*sin(2*q2)*l^2*xc1*xc5 + 2*cos(2*q2)*l^2*xc5^2 - 4*cos(q2)*l*xc1^3 + 4*sin(q2)*l*xc1^2*xc5 - 4*cos(q2)*l*xc1*xc5^2 + 4*sin(q2)*l*xc5^3 - xc1^4 - 2*xc1^2*xc5^2 - xc5^4)^(1/2) - 2*l*xc5))/(l^2 - 2*l*xc1 + xc1^2 + xc5^2 - 2*l^2*cos(q2) + 2*l*xc1*cos(q2) - 2*l*xc5*sin(q2))^2 + (2*(xc1 + l*cos(q2))*(- l^2 + 2*cos(q2)*l*xc1 - 2*sin(q2)*l*xc5 + xc1^2 + xc5^2))/((l^2 - 2*l*xc1 + xc1^2 + xc5^2 - 2*l^2*cos(q2) + 2*l*xc1*cos(q2) - 2*l*xc5*sin(q2))*(3*l^4 + 4*cos(q2)*l^3*xc1 - 4*sin(q2)*l^3*xc5 - 2*cos(2*q2)*l^2*xc1^2 + 4*sin(2*q2)*l^2*xc1*xc5 + 2*cos(2*q2)*l^2*xc5^2 - 4*cos(q2)*l*xc1^3 + 4*sin(q2)*l*xc1^2*xc5 - 4*cos(q2)*l*xc1*xc5^2 + 4*sin(q2)*l*xc5^3 - xc1^4 - 2*xc1^2*xc5^2 - xc5^4)^(1/2))))/((2*l^2*sin(q2) + (3*l^4 + 4*cos(q2)*l^3*xc1 - 4*sin(q2)*l^3*xc5 - 2*cos(2*q2)*l^2*xc1^2 + 4*sin(2*q2)*l^2*xc1*xc5 + 2*cos(2*q2)*l^2*xc5^2 - 4*cos(q2)*l*xc1^3 + 4*sin(q2)*l*xc1^2*xc5 - 4*cos(q2)*l*xc1*xc5^2 + 4*sin(q2)*l*xc5^3 - xc1^4 - 2*xc1^2*xc5^2 - xc5^4)^(1/2) - 2*l*xc5)^2/(l^2 - 2*l*xc1 + xc1^2 + xc5^2 - 2*l^2*cos(q2) + 2*l*xc1*cos(q2) - 2*l*xc5*sin(q2))^2 + 1),                                                                                                                                                                                                                                                                                                                                                                                      (2*((2*l + (2*sin(q2)*l^3 - 2*sin(2*q2)*l^2*xc1 - 2*cos(2*q2)*l^2*xc5 - 2*sin(q2)*l*xc1^2 + 4*cos(q2)*l*xc1*xc5 - 6*sin(q2)*l*xc5^2 + 2*xc1^2*xc5 + 2*xc5^3)/(3*l^4 + 4*cos(q2)*l^3*xc1 - 4*sin(q2)*l^3*xc5 - 2*cos(2*q2)*l^2*xc1^2 + 4*sin(2*q2)*l^2*xc1*xc5 + 2*cos(2*q2)*l^2*xc5^2 - 4*cos(q2)*l*xc1^3 + 4*sin(q2)*l*xc1^2*xc5 - 4*cos(q2)*l*xc1*xc5^2 + 4*sin(q2)*l*xc5^3 - xc1^4 - 2*xc1^2*xc5^2 - xc5^4)^(1/2))/(l^2 - 2*l*xc1 + xc1^2 + xc5^2 - 2*l^2*cos(q2) + 2*l*xc1*cos(q2) - 2*l*xc5*sin(q2)) + ((2*xc5 - 2*l*sin(q2))*(2*l^2*sin(q2) + (3*l^4 + 4*cos(q2)*l^3*xc1 - 4*sin(q2)*l^3*xc5 - 2*cos(2*q2)*l^2*xc1^2 + 4*sin(2*q2)*l^2*xc1*xc5 + 2*cos(2*q2)*l^2*xc5^2 - 4*cos(q2)*l*xc1^3 + 4*sin(q2)*l*xc1^2*xc5 - 4*cos(q2)*l*xc1*xc5^2 + 4*sin(q2)*l*xc5^3 - xc1^4 - 2*xc1^2*xc5^2 - xc5^4)^(1/2) - 2*l*xc5))/(l^2 - 2*l*xc1 + xc1^2 + xc5^2 - 2*l^2*cos(q2) + 2*l*xc1*cos(q2) - 2*l*xc5*sin(q2))^2))/((2*l^2*sin(q2) + (3*l^4 + 4*cos(q2)*l^3*xc1 - 4*sin(q2)*l^3*xc5 - 2*cos(2*q2)*l^2*xc1^2 + 4*sin(2*q2)*l^2*xc1*xc5 + 2*cos(2*q2)*l^2*xc5^2 - 4*cos(q2)*l*xc1^3 + 4*sin(q2)*l*xc1^2*xc5 - 4*cos(q2)*l*xc1*xc5^2 + 4*sin(q2)*l*xc5^3 - xc1^4 - 2*xc1^2*xc5^2 - xc5^4)^(1/2) - 2*l*xc5)^2/(l^2 - 2*l*xc1 + xc1^2 + xc5^2 - 2*l^2*cos(q2) + 2*l*xc1*cos(q2) - 2*l*xc5*sin(q2))^2 + 1),                                                                                                                                                                                                                                                                                                                                                                                                   -(2*((2*l^2*cos(q2) + (2*l*(- sin(q2)*l^2*xc1 - cos(q2)*l^2*xc5 + sin(2*q2)*l*xc1^2 + 2*cos(2*q2)*l*xc1*xc5 - sin(2*q2)*l*xc5^2 + sin(q2)*xc1^3 + cos(q2)*xc1^2*xc5 + sin(q2)*xc1*xc5^2 + cos(q2)*xc5^3))/(3*l^4 + 4*cos(q2)*l^3*xc1 - 4*sin(q2)*l^3*xc5 - 2*cos(2*q2)*l^2*xc1^2 + 4*sin(2*q2)*l^2*xc1*xc5 + 2*cos(2*q2)*l^2*xc5^2 - 4*cos(q2)*l*xc1^3 + 4*sin(q2)*l*xc1^2*xc5 - 4*cos(q2)*l*xc1*xc5^2 + 4*sin(q2)*l*xc5^3 - xc1^4 - 2*xc1^2*xc5^2 - xc5^4)^(1/2))/(l^2 - 2*l*xc1 + xc1^2 + xc5^2 - 2*l^2*cos(q2) + 2*l*xc1*cos(q2) - 2*l*xc5*sin(q2)) + (2*l*(xc5*cos(q2) - l*sin(q2) + xc1*sin(q2))*(2*l^2*sin(q2) + (3*l^4 + 4*cos(q2)*l^3*xc1 - 4*sin(q2)*l^3*xc5 - 2*cos(2*q2)*l^2*xc1^2 + 4*sin(2*q2)*l^2*xc1*xc5 + 2*cos(2*q2)*l^2*xc5^2 - 4*cos(q2)*l*xc1^3 + 4*sin(q2)*l*xc1^2*xc5 - 4*cos(q2)*l*xc1*xc5^2 + 4*sin(q2)*l*xc5^3 - xc1^4 - 2*xc1^2*xc5^2 - xc5^4)^(1/2) - 2*l*xc5))/(l^2 - 2*l*xc1 + xc1^2 + xc5^2 - 2*l^2*cos(q2) + 2*l*xc1*cos(q2) - 2*l*xc5*sin(q2))^2))/((2*l^2*sin(q2) + (3*l^4 + 4*cos(q2)*l^3*xc1 - 4*sin(q2)*l^3*xc5 - 2*cos(2*q2)*l^2*xc1^2 + 4*sin(2*q2)*l^2*xc1*xc5 + 2*cos(2*q2)*l^2*xc5^2 - 4*cos(q2)*l*xc1^3 + 4*sin(q2)*l*xc1^2*xc5 - 4*cos(q2)*l*xc1*xc5^2 + 4*sin(q2)*l*xc5^3 - xc1^4 - 2*xc1^2*xc5^2 - xc5^4)^(1/2) - 2*l*xc5)^2/(l^2 - 2*l*xc1 + xc1^2 + xc5^2 - 2*l^2*cos(q2) + 2*l*xc1*cos(q2) - 2*l*xc5*sin(q2))^2 + 1)];
inv_J =inv(J);
out=inv_J*in;
end

== matlab function controllo_cartesiano/Inerzie ==
  data: parametri input; I output
function I = Inerzie(parametri)
l=parametri(1);
d=parametri(2);
%m1=parametri(3);
ma=parametri(4);


I2 = ma*l^2/4 + 1/12 *ma*l^2;
I5 = I2;
I3 = I2 + 1/12 * ma*d^2 + ma*(d^2/4+l^2/4);
I=[I2;I5;I3];
end
